simulink model "detect_change_complex_test"  (Simulink 8.4)
settings: Solver=ode45  StartTime=0.0  StopTime=10.0  RelTol=1e-3
libraries: simulink x3
settings Model: Creator=arnaud  LastModifiedBy=arnaud
settings DataIOCC: SaveFormat=StructureWithTime

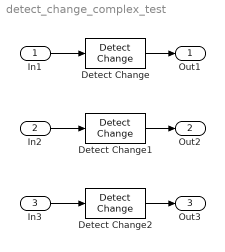
== system detect_change_complex_test ==
  In1 : Inport  PortDimensions=1
      settings: SignalType=complex
  In2 : Inport  Port=2  PortDimensions=5
      settings: SignalType=complex
  In3 : Inport  Port=3  OutDataTypeStr=int8  PortDimensions=[2 3]
      settings: SignalType=complex
  Detect Change : simulink/Logic and Bit Operations/Detect Change  vinit=0  InputProcessing=Inherited  OutDataTypeStr=boolean
  Detect Change1 : simulink/Logic and Bit Operations/Detect Change  vinit=2.5 + 3i  InputProcessing=Inherited  OutDataTypeStr=boolean
  Detect Change2 : simulink/Logic and Bit Operations/Detect Change  vinit=0  InputProcessing=Inherited  OutDataTypeStr=boolean
  Out1 : Outport
  Out2 : Outport  Port=2
  Out3 : Outport  Port=3
  wires:
  Detect Change/1 -> Out1/1
  In1/1 -> Detect Change/1
  Detect Change1/1 -> Out2/1
  In2/1 -> Detect Change1/1
  Detect Change2/1 -> Out3/1
  In3/1 -> Detect Change2/1
